simulink model "spring_damper"  (R2023a)
settings: Solver=VariableStepAuto  StartTime=0.0  StopTime=100  RelTol=1e-3
settings Model: Creator=SHARAYU BOREKAR  LastModifiedBy=SHARAYU BOREKAR

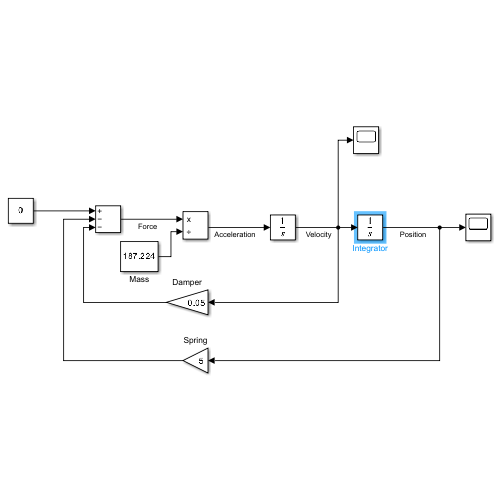
[thumbnail: Simulink's stored preview of the top-level diagram]
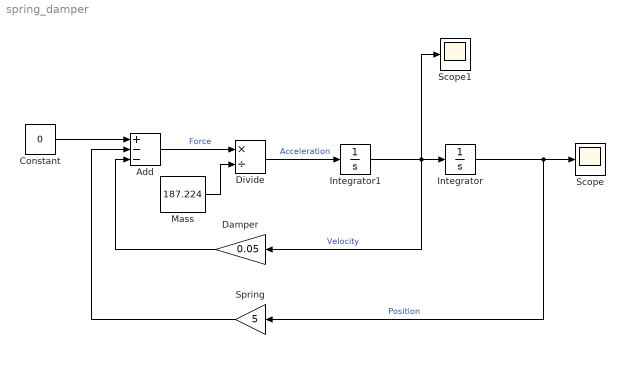
== system spring_damper ==
  Add : Sum  Inputs=+--
  Constant : Constant  Value=0
  Damper : Gain  Gain=0.05
  Divide : Product  Inputs=*/  RndMeth=Zero  SaturateOnIntegerOverflow=on
  Integrator : Integrator  InitialCondition=0.4
  Integrator1 : Integrator
  Mass : Constant  Value=187.224
  Scope : Scope
  Scope1 : Scope
  Spring : Gain  Gain=5
  wires:
  Divide/1 -> Integrator1/1  "Acceleration"
  Add/1 -> Divide/1  "Force"
  Constant/1 -> Add/1
  Integrator1/1 -> Damper/1, Scope1/1, Integrator/1  "Velocity"
  Integrator/1 -> Scope/1, Spring/1  "Position"
  Mass/1 -> Divide/2
  Damper/1 -> Add/3
  Spring/1 -> Add/2
